simulink model "model_2"  (R2023a)
settings: Solver=VariableStepAuto  StartTime=0.0  StopTime=5  FixedStep=0.0001  RelTol=1e-3
values from neighbouring files (symbols this model uses):
  A = [0 1; -4 0]    [data_2.m]
  B = [0;0]    [data_2.m]
  C = [1 0]    [data_2.m]
  sin_dt1 = 0.2    [data_2.m]
  sin_dt2 = 1/30    (= 0.0333333333333)    [data_2.m]
  sin_dt3 = 0.01    [data_2.m]
  system_disc1 = c2d(system_contin, sin_dt1)    [data_2.m]
  system_disc2 = c2d(system_contin, sin_dt2)    [data_2.m]
  system_disc3 = c2d(system_contin, sin_dt3)    [data_2.m]
settings Model: Creator=TheMix  LastModifiedBy=TheMix

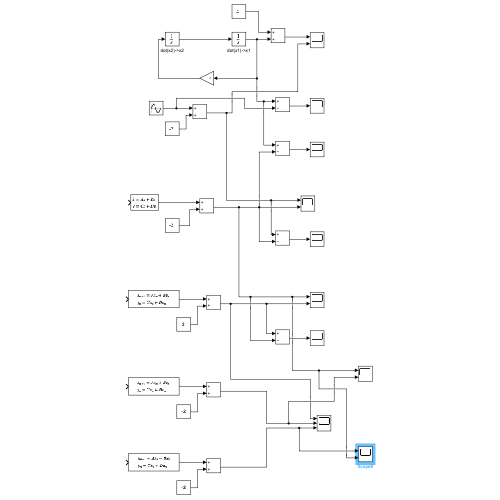
[thumbnail: Simulink's stored preview of the top-level diagram]
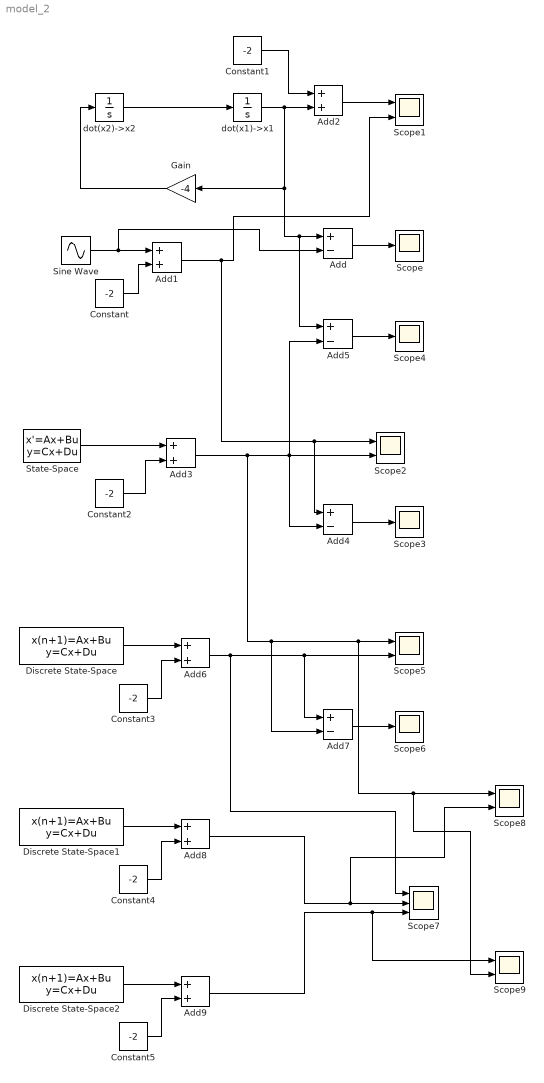
== system model_2 ==
  Add{,4..5,7} (4 alike) : Sum  Inputs=+-
  Add{1..3,6,8..9} (6 alike) : Sum
  Constant{,1..5} (6 alike) : Constant  Value=-2
  Discrete State-Space : DiscreteStateSpace  A=system_disc1.A  B=system_disc1.B  C=system_disc1.C  D=system_disc1.D  InitialCondition=[2*sin(pi/3); 2]  SampleTime=sin_dt1
  Discrete State-Space1 : DiscreteStateSpace  A=system_disc2.A  B=system_disc2.B  C=system_disc2.C  D=system_disc2.D  InitialCondition=[2*sin(pi/3); 2]  SampleTime=sin_dt2
  Discrete State-Space2 : DiscreteStateSpace  A=system_disc3.A  B=system_disc3.B  C=system_disc3.C  D=system_disc3.D  InitialCondition=[2*sin(pi/3); 2]  SampleTime=sin_dt3
  Gain : Gain  Gain=-4
  Scope{,3..4,6} (4 alike) : Scope
  Scope{1..2,5,8..9} (5 alike) : Scope  NumInputPorts=2
  Scope7 : Scope  NumInputPorts=3
  Sine Wave : Sin  Amplitude=2  Frequency=2  Phase=pi/3  SampleTime=0
  State-Space : StateSpace  A=A  B=B  C=C  D=0  InitialCondition=[2*sin(pi/3); 2]
  dot(x1)->x1 : Integrator  InitialCondition=2*sin(pi/3)
  dot(x2)->x2 : Integrator  InitialCondition=2
  wires:
  dot(x2)->x2/1 -> dot(x1)->x1/1
  Gain/1 -> dot(x2)->x2/1
  Add/1 -> Scope/1
  Add1/1 -> Add4/1, Scope2/1, Scope1/2
  Sine Wave/1 -> Add/2, Add1/1
  Constant/1 -> Add1/2
  Add2/1 -> Scope1/1
  dot(x1)->x1/1 -> Add5/1, Add/1, Gain/1, Add2/2
  Constant1/1 -> Add2/1
  Constant2/1 -> Add3/2
  Add3/1 -> Add7/2, Scope9/2, Scope8/1, Scope5/1, Add4/2, Add5/2, Scope2/2
  State-Space/1 -> Add3/1
  Add4/1 -> Scope3/1
  Add5/1 -> Scope4/1
  Discrete State-Space/1 -> Add6/1
  Add6/1 -> Scope7/1, Add7/1, Scope5/2
  Constant3/1 -> Add6/2
  Add7/1 -> Scope6/1
  Constant4/1 -> Add8/2
  Discrete State-Space1/1 -> Add8/1
  Discrete State-Space2/1 -> Add9/1
  Constant5/1 -> Add9/2
  Add9/1 -> Scope9/1, Scope7/3
  Add8/1 -> Scope8/2, Scope7/2
